simulink model "verify_Electric_Heater_Ctrl_mdl"  (R2018b)
settings: Solver=ode45  StartTime=0  StopTime=1200  MaxStep=60  RelTol=1e-3  EnableMultiTasking=on
libraries: carnot x3
settings Model: Creator=drhf  LastModifiedBy=drhf
settings DataIOCC: SaveFormat=Array  SignalLoggingSaveFormat=ModelDataLogs
settings OptimizationCC: ExpressionDepthLimit=2147483647  LifeSpan=inf
settings DebuggingCC: UnderspecifiedInitializationDetection=Classic  MergeDetectMultiDrivingBlocksExec=none  SolverPrmCheckMsg=warning  FcnCallInpInsideContextMsg=warning  StateNameClashWarn=warning  SFUnexpectedBacktrackingDiag=warning  SFNoUnconditionalDefaultTransitionDiag=warning  SFExecutionAtInitializationDiag=none
settings HardwareCC: ProdBitPerPointer=32  ProdBitPerSizeT=32  ProdBitPerPtrDiffT=32  ProdLargestAtomicFloat=None  ProdIntDivRoundTo=Undefined  ProdEndianess=Unspecified  ProdWordSize=32  ProdHWDeviceType=32-bit Generic
settings ModelReferenceCC: PropagateSignalLabelsOutOfModel=off
settings SFSimCC: SimUseLocalCustomCode=off
settings RTWCC: RTWUseLocalCustomCode=off
settings CodeAppCC: StateflowObjectComments=on
settings GRTTargetCC: TargetLangStandard=C89/C90 (ANSI)  GeneratePreprocessorConditionals=Disable all  CombineOutputUpdateFcns=off  GRTInterface=on
settings ConfigComp: CovMetricSettings=dw  CovHtmlReporting=on  CovSaveCumulativeToWorkspaceVar=on  CovSaveSingleToWorkspaceVar=on  CovExternalEMLEnable=off

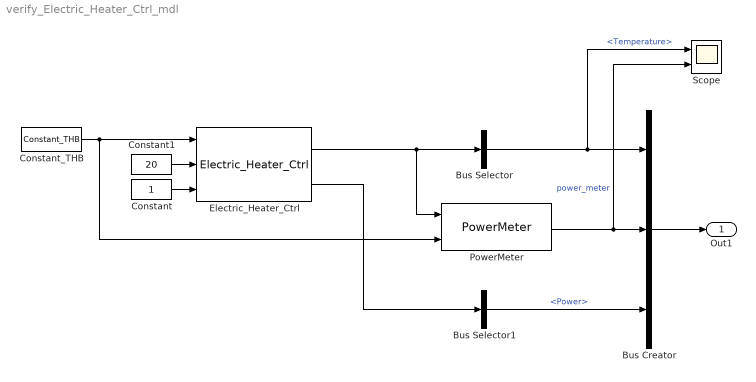
== system verify_Electric_Heater_Ctrl_mdl ==
  Bus Creator : BusCreator  Inputs=3
  Bus Selector : BusSelector  OutputSignals=Temperature
  Bus Selector1 : BusSelector  OutputSignals=Power
  Constant : Constant
  Constant1 : Constant  Value=20
  Constant_THB : carnot/Source/Simple/Constant_THB  t=40  mdot=500/3600  p=1e5  mID=No Pressure Drop  fluid=Water  mix=0  mix2=0  mix3=0  dia=0.02  hgt=0
      settings: SourceProductName=Carnot
  Electric_Heater_Ctrl : carnot/Source/Boiler/Electric_Heater_Ctrl  power=1000  UA=1  mcp=3*4182  Tini=40
      settings: SourceProductName=Carnot
  PowerMeter : carnot/Control/PowerMeter
      settings: SourceProductName=Carnot
  Scope : Scope  NumInputPorts=2
  Out1 : Outport
  wires:
  Bus Creator/1 -> Out1/1
  Bus Selector/1 -> Scope/1, Bus Creator/1  "<Temperature>"
  PowerMeter/1 -> Scope/2, Bus Creator/2  "power_meter"
  Constant/1 -> Electric_Heater_Ctrl/3
  Constant_THB/1 -> PowerMeter/2, Electric_Heater_Ctrl/1
  Electric_Heater_Ctrl/1 -> Bus Selector/1, PowerMeter/1
  Electric_Heater_Ctrl/2 -> Bus Selector1/1
  Bus Selector1/1 -> Bus Creator/3  "<Power>"
  Constant1/1 -> Electric_Heater_Ctrl/2
